simulink model "validation_block"  (R2025b)
settings: Solver=FixedStepDiscrete  StartTime=0  StopTime=1  FixedStep=1e-4  RelTol=1e-3
settings Model: Creator=Ashwin  LastModifiedBy=Ashwin
settings DataIOCC: SaveFormat=StructureWithTime

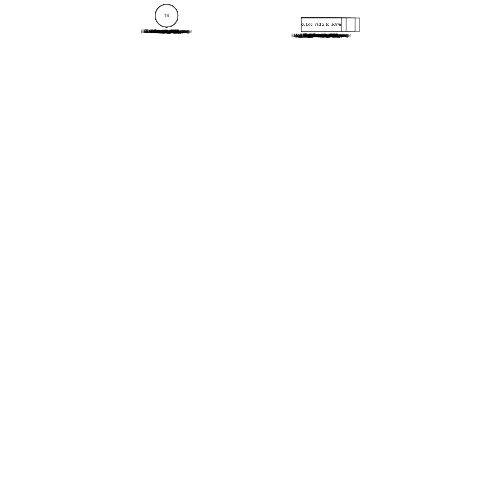
[thumbnail: Simulink's stored preview of the top-level diagram]
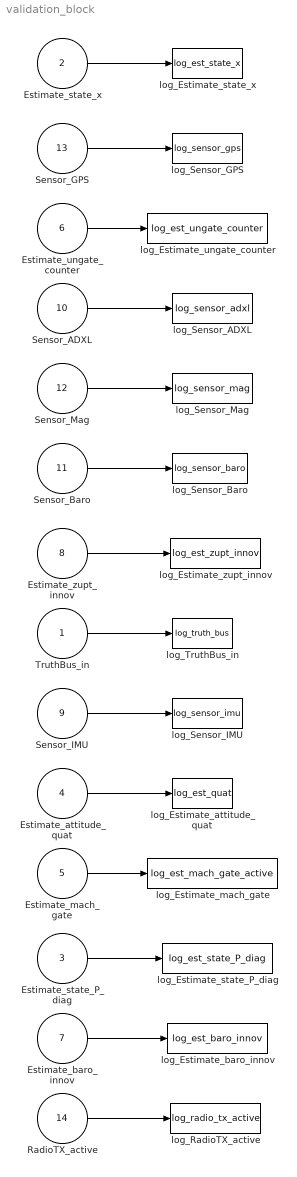
== system validation_block ==
  TruthBus_in : Inport
  Estimate_state_x : Inport  Port=2
  Estimate_state_P_diag : Inport  Port=3
  Estimate_attitude_quat : Inport  Port=4
  Estimate_mach_gate : Inport  Port=5
  Estimate_ungate_counter : Inport  Port=6
  Estimate_baro_innov : Inport  Port=7
  Estimate_zupt_innov : Inport  Port=8
  Sensor_IMU : Inport  Port=9
  Sensor_ADXL : Inport  Port=10
  Sensor_Baro : Inport  Port=11
  Sensor_Mag : Inport  Port=12
  Sensor_GPS : Inport  Port=13
  RadioTX_active : Inport  Port=14
  log_Estimate_attitude_quat : ToWorkspace  VariableName=log_est_quat  SaveFormat=Structure With Time  SampleTime=-1
  log_Estimate_baro_innov : ToWorkspace  VariableName=log_est_baro_innov  SaveFormat=Structure With Time  SampleTime=-1
  log_Estimate_mach_gate : ToWorkspace  VariableName=log_est_mach_gate_active  SaveFormat=Structure With Time  SampleTime=-1
  log_Estimate_state_P_diag : ToWorkspace  VariableName=log_est_state_P_diag  SaveFormat=Structure With Time  SampleTime=-1
  log_Estimate_state_x : ToWorkspace  VariableName=log_est_state_x  SaveFormat=Structure With Time  SampleTime=-1
  log_Estimate_ungate_counter : ToWorkspace  VariableName=log_est_ungate_counter  SaveFormat=Structure With Time  SampleTime=-1
  log_Estimate_zupt_innov : ToWorkspace  VariableName=log_est_zupt_innov  SaveFormat=Structure With Time  SampleTime=-1
  log_RadioTX_active : ToWorkspace  VariableName=log_radio_tx_active  SaveFormat=Structure With Time  SampleTime=-1
  log_Sensor_ADXL : ToWorkspace  VariableName=log_sensor_adxl  SaveFormat=Structure With Time  SampleTime=-1
  log_Sensor_Baro : ToWorkspace  VariableName=log_sensor_baro  SaveFormat=Structure With Time  SampleTime=-1
  log_Sensor_GPS : ToWorkspace  VariableName=log_sensor_gps  SaveFormat=Structure With Time  SampleTime=-1
  log_Sensor_IMU : ToWorkspace  VariableName=log_sensor_imu  SaveFormat=Structure With Time  SampleTime=-1
  log_Sensor_Mag : ToWorkspace  VariableName=log_sensor_mag  SaveFormat=Structure With Time  SampleTime=-1
  log_TruthBus_in : ToWorkspace  VariableName=log_truth_bus  SaveFormat=Structure With Time  SampleTime=-1
  wires:
  Estimate_state_x/1 -> log_Estimate_state_x/1
  TruthBus_in/1 -> log_TruthBus_in/1
  RadioTX_active/1 -> log_RadioTX_active/1
  Sensor_GPS/1 -> log_Sensor_GPS/1
  Sensor_Mag/1 -> log_Sensor_Mag/1
  Sensor_Baro/1 -> log_Sensor_Baro/1
  Estimate_state_P_diag/1 -> log_Estimate_state_P_diag/1
  Estimate_mach_gate/1 -> log_Estimate_mach_gate/1
  Estimate_attitude_quat/1 -> log_Estimate_attitude_quat/1
  Estimate_ungate_counter/1 -> log_Estimate_ungate_counter/1
  Estimate_baro_innov/1 -> log_Estimate_baro_innov/1
  Sensor_IMU/1 -> log_Sensor_IMU/1
  Sensor_ADXL/1 -> log_Sensor_ADXL/1
  Estimate_zupt_innov/1 -> log_Estimate_zupt_innov/1
